simulink model "multi_in_state_out_1t_2sint"  (R2021b)
settings: Solver=VariableStepAuto  StartTime=0.0  StopTime=10.0  RelTol=1e-3
settings Model: Creator=den  LastModifiedBy=den

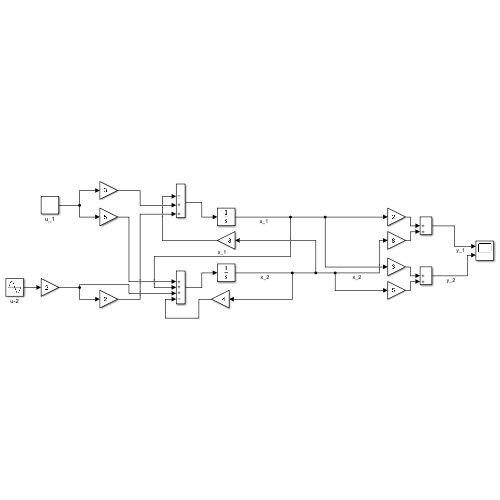
[thumbnail: Simulink's stored preview of the top-level diagram]
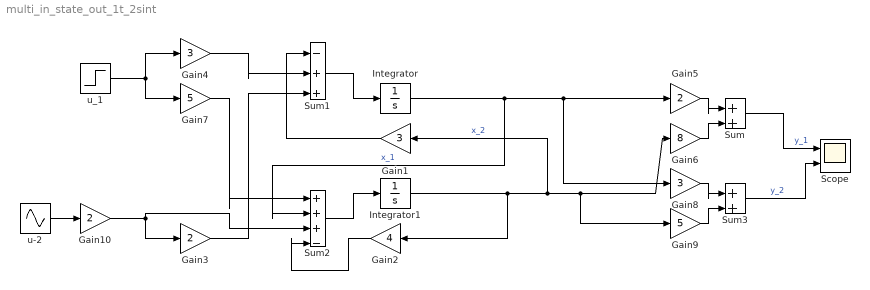
== system multi_in_state_out_1t_2sint ==
  Gain1 : Gain  Gain=3
  Gain10 : Gain  Gain=2
  Gain2 : Gain  Gain=4
  Gain3 : Gain  Gain=2
  Gain4 : Gain  Gain=3
  Gain5 : Gain  Gain=2
  Gain6 : Gain  Gain=8
  Gain7 : Gain  Gain=5
  Gain8 : Gain  Gain=3
  Gain9 : Gain  Gain=5
  Integrator : Integrator
  Integrator1 : Integrator
  Scope : Scope  NumInputPorts=2
  Sum : Sum  Inputs=|++
  Sum1 : Sum  Inputs=|-++
  Sum2 : Sum  Inputs=|+++-
  Sum3 : Sum  Inputs=|++
  u-2 : Sin  SampleTime=0
  u_1 : Step  SampleTime=0
  wires:
  Sum1/1 -> Integrator/1
  Sum2/1 -> Integrator1/1
  Integrator/1 -> Gain8/1, Gain5/1, Sum2/2  "x_1"
  Integrator1/1 -> Gain1/1, Gain9/1, Gain6/1, Gain2/1  "x_2"
  u_1/1 -> Gain7/1, Gain4/1
  u-2/1 -> Gain10/1
  Gain4/1 -> Sum1/2
  Gain3/1 -> Sum1/3
  Gain1/1 -> Sum1/1
  Gain2/1 -> Sum2/4
  Gain7/1 -> Sum2/1
  Gain5/1 -> Sum/1
  Gain6/1 -> Sum/2
  Sum/1 -> Scope/1  "y_1"
  Gain8/1 -> Sum3/1
  Gain9/1 -> Sum3/2
  Sum3/1 -> Scope/2  "y_2"
  Gain10/1 -> Sum2/3, Gain3/1
